simulink model "ex_ass3_2022a"  (R2022a)
settings: Solver=FixedStepAuto  StartTime=0.0  StopTime=inf  FixedStep=0.05  RelTol=1e-3
model workspace (MAT data in the model file):
  SL_ROS_VariableLengthArrays_MaxSizes.CommonInfo.ArrayTruncateAction = 'EmitWarning'
  SL_ROS_VariableLengthArrays_MaxSizes.MsgTypeMap = containers.Map
  SL_ROS_VariableLengthArrays_MaxSizes.MsgTypeMap.serialization.keys = {'sensor_msgs/Image'}
  SL_ROS_VariableLengthArrays_MaxSizes.MsgTypeMap.serialization.values{1}(1).PropertyName = 'Data'
  SL_ROS_VariableLengthArrays_MaxSizes.MsgTypeMap.serialization.values{1}(1).DataType = 'uint8'
  SL_ROS_VariableLengthArrays_MaxSizes.MsgTypeMap.serialization.values{1}(1).MaxLength = 921600
  SL_ROS_VariableLengthArrays_MaxSizes.MsgTypeMap.serialization.values{1}(2).PropertyName = 'Encoding'
  SL_ROS_VariableLengthArrays_MaxSizes.MsgTypeMap.serialization.values{1}(2).DataType = 'uint8'
  SL_ROS_VariableLengthArrays_MaxSizes.MsgTypeMap.serialization.values{1}(2).MaxLength = 128
  SL_ROS_VariableLengthArrays_MaxSizes.MsgTypeMap.serialization.uniformity = 0
  SL_ROS_VariableLengthArrays_MaxSizes.MsgTypeMap.serialization.keyType = 'char'
  SL_ROS_VariableLengthArrays_MaxSizes.MsgTypeMap.serialization.valueType = 'any'
values from neighbouring files (symbols this model uses):
  blueMax = 120    [Ass3_ex.m]
  darkMin = 30    [Ass3_ex.m]
undefined symbols (not defined in the file or in its folder): gray, Rec, SDTV
libraries: robotlib x2, visionstatistics x1, visionconversions x1, visiontextngfix x1, simulink x1
settings Model: Creator=raibuntu  LastModifiedBy=jacopo
settings OptimizationCC: EnhancedBackFolding=on  PassReuseOutputArgsAs=Individual arguments  ZeroExternalMemoryAtStartup=off  ZeroInternalMemoryAtStartup=off  MaxStackSize=64  OptimizeBlockOrder=speed  DifferentSizesBufferReuse=on  OptimizationCustomize=off  EfficientTunableParamExpr=on
settings DebuggingCC: ParameterTunabilityLossMsg=error
settings HardwareCC: ProdBitPerPointer=32  ProdBitPerSizeT=32  ProdBitPerPtrDiffT=32  ProdLargestAtomicFloat=None  ProdIntDivRoundTo=Undefined  ProdEndianess=Unspecified  ProdWordSize=32  ProdHWDeviceType=Generic->Unspecified (assume 32-bit Generic)
settings ModelReferenceCC: EnableRefExpFcnMdlSchedulingChecks=off
settings SFSimCC: MATLABDynamicMemAlloc=off
settings RTWCC: SystemTargetFile=ert.tlc  HardwareBoard=Robot Operating System (ROS)  TLCOptions="-aInlineSetEventsForThisBaseRateFcn=TLC_FALSE -aSuppressMultiTaskScheduler=TLC_FALSE  -aRateBasedStepFcn=0"  TemplateMakefile=ert_default_tmf  Toolchain=Catkin  TargetLang=C++
settings CodeAppCC: ForceParamTrailComments=on  IgnoreCustomStorageClasses=off  OperatorAnnotations=on  SimulinkDataObjDesc=on  SFDataObjDesc=on  InsertBlockDesc=on

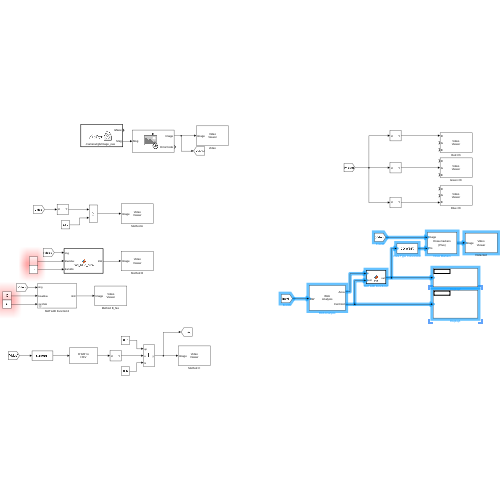
[thumbnail: Simulink's stored preview of the top-level diagram]
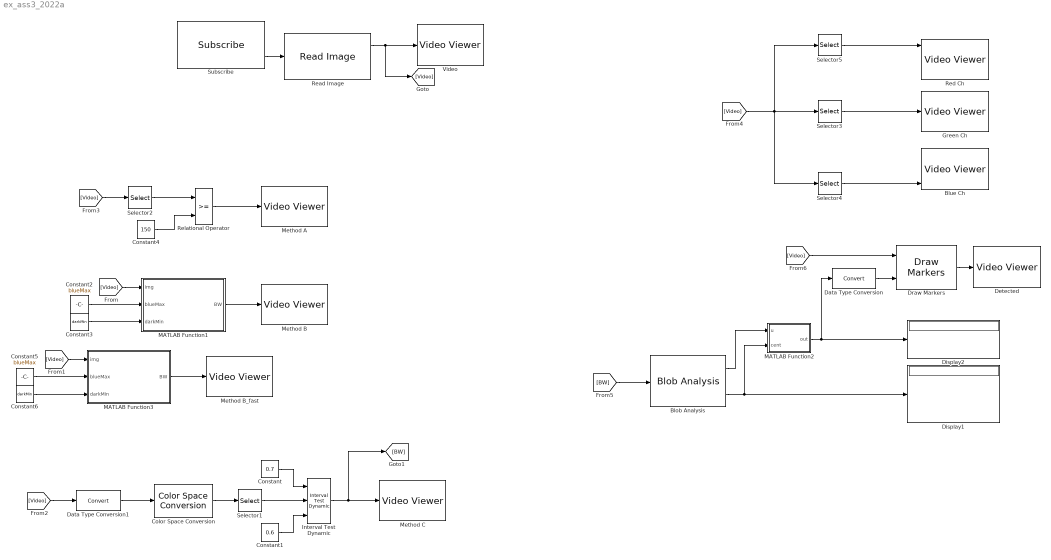
== system ex_ass3_2022a ==
  Blob Analysis : visionstatistics/Blob Analysis  Tag=vipblks_row_conv  area=on  centroid=on  bBox=off  majorAxis=off  minorAxis=off  angle=off  eccentricity=off  equivDiameterSq=off  extent=off  perimeter=off  outDT=double  conn=8  isLabel=off  maxBlobs=5  warnIfNumBlobsExceeded=on  isCount=off  useMinArea=off  minArea=0  useMaxArea=off  maxArea=intmax('uint32')  excludeBorderBlob=off  isOutVarDim=off  isFill=on  fillValues=-1  roundingMode=Floor  overflowMode=off  prodOutputMode=Binary point scaling  prodOutputWordLength=32  prodOutputFracLength=16  accumMode=Binary point scaling  accumWordLength=32  accumFracLength=0  outputMode=Binary point scaling  outputWordLength=32  outputFracLength=16  firstCoeffMode=Binary point scaling  firstCoeffWordLength=16  firstCoeffFracLength=14  secondCoeffMode=Binary point scaling  secondCoeffWordLength=32  secondCoeffFracLength=16
  Blue Ch : VideoViewer  imagePorts=separate color signals  FigPos=[295 869 802 390]
  Color Space Conversion : visionconversions/Color Space  Conversion  conversion=Obsolete  conversionActive=R'G'B' to HSV  wp_str=D65  rec=Rec. 601 (SDTV)  sys=1125/60/2:1  imagePorts=One multidimensional signal
  Constant : Constant  Value=0.7
  Constant1 : Constant  Value=0.6
  Constant2 : Constant  Value=blueMax
  Constant3 : Constant  Value=darkMin
  Constant4 : Constant  Value=150  OutDataTypeStr=uint8
  Constant5 : Constant  Value=blueMax
  Constant6 : Constant  Value=darkMin
  Data Type Conversion : DataTypeConversion  SaturateOnIntegerOverflow=off  RndMeth=Floor
  Data Type Conversion1 : DataTypeConversion  SaturateOnIntegerOverflow=off  RndMeth=Floor
  Detected : VideoViewer  colormapValue=gray(256)  FigPos=[797 832 589 391]
  Display1 : Display
  Display2 : Display
  Draw Markers : visiontextngfix/Draw Markers  shape=Plus  size=30  fill=off  fillClrSource=Specify via dialog  display=User-specified value  intensity=200  color=[255 0 0]  opacity=0.6  viewport=Entire image  antialiasing=off  inType=Obsolete  imagePorts=One multidimensional signal  roundingMode=Floor  overflowMode=off  memoryMode=Specify word length  memoryWordLength=16  memoryFracLength=15  prodOutputMode=Binary point scaling  prodOutputWordLength=32  prodOutputFracLength=14
      settings: SourceProductBaseCode=VP
  Green Ch : VideoViewer  imagePorts=separate color signals  FigPos=[995 785 782 404]
  Interval Test Dynamic : simulink/Logic and Bit Operations/Interval Test Dynamic  IntervalClosedRight=on  IntervalClosedLeft=on  OutDataTypeStr=boolean
      settings: SourceProductBaseCode=SL
  MATLAB Function1 : MATLAB Function  TreatAsAtomicUnit=on
  MATLAB Function2 : MATLAB Function  TreatAsAtomicUnit=on
  MATLAB Function3 : Subsystem
      mask help: Simulink:masks:GenSFuncDesc_MD
      mask Help: eval('feval(''rtwprivate'',''rtwhelpview'',''rtw_sfcn_block'')');
  Method A : VideoViewer  colormapValue=gray(256)  FigPos=[1168 765 555 411]
  Method B : VideoViewer  colormapValue=gray(256)  FigPos=[879 781 690 412]
  Method B_fast : VideoViewer  colormapValue=gray(256)  FigPos=[264 768 596 398]
  Method C : VideoViewer  colormapValue=gray(256)  FigPos=[1101 806 587 411]
  Read Image : robotlib/Read Image  MaximumImageSize=[480, 640]  ImageEncoding=rgb8  ShowAlphaOutput=off  ShowErrorCodeOutput=on  VariableSizeOutputs=off
      settings: SourceProductBaseCode=RR
  Red Ch : VideoViewer  imagePorts=separate color signals  FigPos=[1013 930 782 404]
  Relational Operator : RelationalOperator  OutDataTypeStr=boolean  RndMeth=Simplest  InputSameDT=off
  Selector1 : Selector  NumberOfDimensions=3  InputPortWidth=3  IndexOptions=Index vector (dialog),Index vector (dialog),Index vector (dialog)  Indices=[1:480],[1:640],1  OutputSizes=1,1,1
  Selector2 : Selector  NumberOfDimensions=3  InputPortWidth=3  IndexOptions=Index vector (dialog),Index vector (dialog),Index vector (dialog)  Indices=[1:480],[1:640],3  OutputSizes=1,1,1
  Selector3 : Selector  NumberOfDimensions=3  InputPortWidth=3  IndexOptions=Index vector (dialog),Index vector (dialog),Index vector (dialog)  Indices=[1:480],[1:640],2  OutputSizes=1,1,1
  Selector4 : Selector  NumberOfDimensions=3  InputPortWidth=3  IndexOptions=Index vector (dialog),Index vector (dialog),Index vector (dialog)  Indices=[1:480],[1:640],3  OutputSizes=1,1,1
  Selector5 : Selector  NumberOfDimensions=3  InputPortWidth=3  IndexOptions=Index vector (dialog),Index vector (dialog),Index vector (dialog)  Indices=[1:480],[1:640],1  OutputSizes=1,1,1
  Subscribe : robotlib/Subscribe  topicSource=Select from ROS network  topic=/camera/rgb/image_raw  messageType=sensor_msgs/Image  SampleTime=-1  legacyBusStruct=off  messageQueueLength=1
  Video : VideoViewer  colormapValue=gray(256)  FigPos=[230 860 666 466]
  wires:
  Constant2/1 -> MATLAB Function1/2(blueMax)
  Constant3/1 -> MATLAB Function1/3(darkMin)
  MATLAB Function1/1(BW) -> Method B/1
  Blob Analysis/2 -> Display1/1, MATLAB Function2/2(cent)
  Blob Analysis/1 -> MATLAB Function2/1(u)
  MATLAB Function2/1(out) -> Data Type Conversion/1, Display2/1
  Draw Markers/1 -> Detected/1
  Data Type Conversion/1 -> Draw Markers/2
  Color Space Conversion/1 -> Selector1/1
  Data Type Conversion1/1 -> Color Space Conversion/1
  Subscribe/2 -> Read Image/1
  Selector1/1 -> Interval Test Dynamic/2
  Constant/1 -> Interval Test Dynamic/1
  Constant1/1 -> Interval Test Dynamic/3
  Selector2/1 -> Relational Operator/1
  Constant4/1 -> Relational Operator/2
  Relational Operator/1 -> Method A/1
  Selector3/1 -> Green Ch/2
  Selector4/1 -> Blue Ch/3
  Constant6/1 -> MATLAB Function3/3(darkMin)
  Constant5/1 -> MATLAB Function3/2(blueMax)
  MATLAB Function3/1(BW) -> Method B_fast/1
  Read Image/1 -> [Video], Video/1
  [Video] -> MATLAB Function1/1(img)
  [Video] -> MATLAB Function3/1(img)
  Interval Test Dynamic/1 -> [BW], Method C/1
  [Video] -> Data Type Conversion1/1
  [Video] -> Selector2/1
  Selector5/1 -> Red Ch/1
  [Video] -> Selector4/1, Selector5/1, Selector3/1
  [BW] -> Blob Analysis/1
  [Video] -> Draw Markers/1

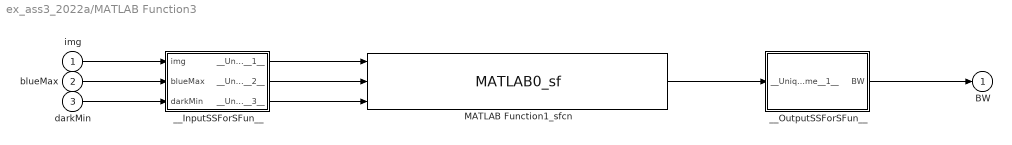
== system ex_ass3_2022a/MATLAB Function3 ==
  img : Inport
  blueMax : Inport  Port=2
  darkMin : Inport  Port=3
  MATLAB Function1_sfcn : S-Function  FunctionName=MATLAB0_sf  SFunctionModules=""  SFunctionDeploymentMode=off  EnableBusSupport=off  mask{rtw_sf_name=MATLAB0_sf, showVar=off}
      mask prompts: rtw_sf_name "Simulink:masks:GenSFuncName_MP"; showVar "Simulink:masks:GenSFuncShowModuleList_MP"
      mask help: Simulink:masks:GenSFuncDesc_MD
      mask init:
      | displist = '';
      | if ~strcmp(get_param(gcb, 'FunctionName'), rtw_sf_name);
      |   set_param(gcb, 'FunctionName', rtw_sf_name);
      | end
      | % Check if we are generating code
      | rtw_mode = false;
      | if strcmpi(get_param(bdroot(gcb),'SimulationStatus'),'Initializing')
      | 	rtw_mode = strcmpi(get_param(bdroot(gcb),'BuildingRTWCode'),'on') && ...
      | 		~strcmpi(get_param(bdroot(gcb),'TargetStyle'),'SimulationTarget');
      | end
      | if showVar || rtw_mode
      | 	if exist('rtwsfunc') == 2 | exist('rtwsfunc') == 6
      | 		tmplist = rtwsfunc(rtw_sf_name,gcb);
      | 		tmplist = DAStudio.message('Simulink:masks:GenSFuncListOfModules_IC', tmplist);
      | 	elseif showVar
      | 		tmplist1 = DAStudio.message('Simulink:masks:GenSFuncListOfModules_IC', '');
      |         tmplist2 = DAStudio.message('Simulink:masks:GenSFuncNotLicensed_IC');
      |         tmplist = [tmplist1 tmplist2];
      |  	end
      | end
      | if showVar
      |   displist = tmplist;
      | end
      settings: CopyFcn=|
      | if ~strcmp(get_param(gcb,'Linkstatus'),'none') && ...
      | ~strcmp(get_param(gcb,'Linkstatus'),'implicit')
      |   set_param(gcb,'LinkStatus','none');
      | end
      mask Help: eval('feval(''rtwprivate'',''rtwhelpview'',''rtw_sfcn_block'')');
      mask Display:
      | port_label('input',1,'img');
      | port_label('input',2,'blueMax');
      | port_label('input',3,'darkMin');
      | port_label('output',1,'BW');
  __InputSSForSFun__ : Subsystem
  __OutputSSForSFun__ : Subsystem
  BW : Outport
  wires:
  img/1 -> __InputSSForSFun__/1(img)
  blueMax/1 -> __InputSSForSFun__/2(blueMax)
  darkMin/1 -> __InputSSForSFun__/3(darkMin)
  __InputSSForSFun__/1(__UniqueOutportName__1__) -> MATLAB Function1_sfcn/1
  __InputSSForSFun__/2(__UniqueOutportName__2__) -> MATLAB Function1_sfcn/2
  __InputSSForSFun__/3(__UniqueOutportName__3__) -> MATLAB Function1_sfcn/3
  MATLAB Function1_sfcn/1 -> __OutputSSForSFun__/1(__UniqueInportName__1__)
  __OutputSSForSFun__/1(BW) -> BW/1

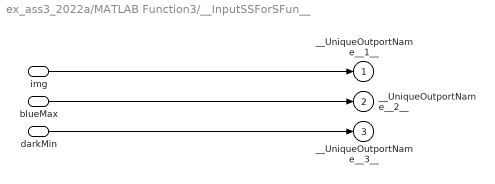
== system ex_ass3_2022a/MATLAB Function3/__InputSSForSFun__ ==
  img : Inport
  blueMax : Inport  Port=2
  darkMin : Inport  Port=3
  __UniqueOutportName__1__ : Outport
  __UniqueOutportName__2__ : Outport  Port=2
  __UniqueOutportName__3__ : Outport  Port=3
  wires:
  img/1 -> __UniqueOutportName__1__/1
  blueMax/1 -> __UniqueOutportName__2__/1
  darkMin/1 -> __UniqueOutportName__3__/1

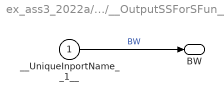
== system ex_ass3_2022a/MATLAB Function3/__OutputSSForSFun__ ==
  __UniqueInportName__1__ : Inport
  BW : Outport
  wires:
  __UniqueInportName__1__/1 -> BW/1  "BW"

== matlab function ex_ass3_2022a/MATLAB Function2 ==
  data: u input; cent input; out output
function out  = fcn(u,cent)

[~,i] = max(u);

if ~isempty(i)
    out=cent(i,:);
else 
    out=[0,0];
end

== matlab function ex_ass3_2022a/MATLAB Function1 ==
  data: img input; BW output; blueMax input; darkMin input
function BW = find_blue_area(img,blueMax,darkMin)

blueImg = img(:,:,1)/2 + img(:,:,2)/2 - img(:,:,3)/2;
    blueThresh = blueImg < blueMax;
    darkIso = -img(:,:,1)/2 - img(:,:,2)/2 + 3*img(:,:,3) - 2*rgb2gray(img);
    darkThresh = darkIso > darkMin;
    BW = blueThresh & darkThresh;
% BW=img;
